simulink model "q3_week1"  (R2024b)
settings: Solver=VariableStepAuto  StartTime=0.0  StopTime=10.0  RelTol=1e-3
settings Model: Creator=Sagar  LastModifiedBy=Sagar

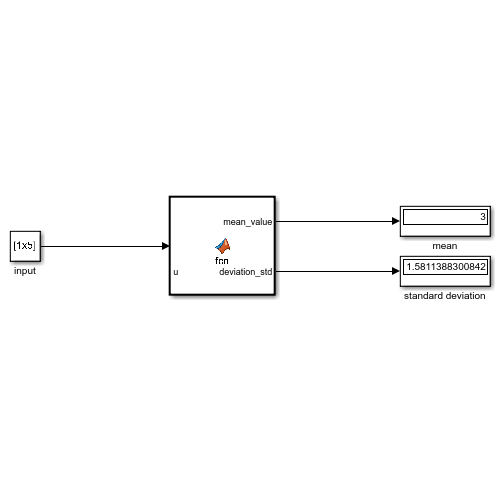
[thumbnail: Simulink's stored preview of the top-level diagram]
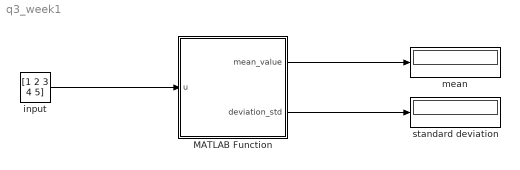
== system q3_week1 ==
  MATLAB Function : MATLAB Function  TreatAsAtomicUnit=on
  input : Constant  Value=[1 2 3 4 5]
  mean : Display
      settings: Format=decimal (Stored Integer)
  standard deviation : Display
      settings: Format=decimal (Stored Integer)
  wires:
  input/1 -> MATLAB Function/1(u)
  MATLAB Function/1(mean_value) -> mean/1
  MATLAB Function/2(deviation_std) -> standard deviation/1

== matlab function q3_week1/MATLAB Function ==
  data: u input; mean_value output; deviation_std output
function [mean_value, deviation_std] = fcn(u)
% MATLAB Function for Simulink: Computes mean and standard deviation
% Ensure the output variables are properly defined

mean_value = mean(u);
deviation_std = std(u);

end
